simulink model "ExampleModel"  (R2019a)
settings: Solver=VariableStepAuto  StartTime=0.0  StopTime=10.0  RelTol=1e-3  EnableMultiTasking=on
values from neighbouring files (symbols this model uses):
  Param_Mus = Library_mtu_simulink_mtu_standard_parameters(Param_Mus)    [init_muscle.m]
libraries: Library_mtu_simulink x2, simulink x1
settings Model: Creator=danielhaeufle  LastModifiedBy=danielhaeufle
settings DataIOCC: ReturnWorkspaceOutputs=off
settings OptimizationCC: LifeSpan=inf
settings DebuggingCC: SFUnexpectedBacktrackingDiag=warning  SFNoUnconditionalDefaultTransitionDiag=warning  ArithmeticOperatorsInVariantConditions=warning
settings SFSimCC: SimUseLocalCustomCode=off
settings RTWCC: RTWUseLocalCustomCode=off
settings CodeAppCC: StateflowObjectComments=on
settings GRTTargetCC: TargetLangStandard=C89/C90 (ANSI)  GeneratePreprocessorConditionals=Disable all
settings ConfigComp: CovMetricSettings=dw  CovHtmlReporting=on  CovSaveCumulativeToWorkspaceVar=on  CovSaveSingleToWorkspaceVar=on  CovExternalEMLEnable=off

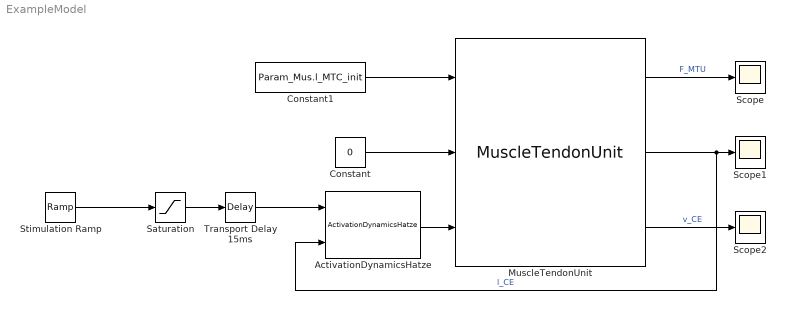
== system ExampleModel ==
  ActivationDynamicsHatze : Library_mtu_simulink/ActivationDynamicsHatze  Act_Param=Param_Mus.ActDyn  Mus_Param=Param_Mus
  Constant : Constant  Value=0
  Constant1 : Constant  Value=Param_Mus.l_MTC_init
  MuscleTendonUnit : Library_mtu_simulink/MuscleTendonUnit  Mus_Param=Param_Mus
  Saturation : Saturate  UpperLimit=1  LowerLimit=0.001
  Scope : Scope
  Scope1 : Scope
  Scope2 : Scope
  Stimulation Ramp : simulink/Sources/Ramp  slope=0.1  start=0  InitialOutput=0
  Transport Delay 15ms : TransportDelay  DelayTime=0.015  InitialOutput=Param_Mus.ActDyn.u_init
  wires:
  Saturation/1 -> Transport Delay 15ms/1
  ActivationDynamicsHatze/1 -> MuscleTendonUnit/3
  Transport Delay 15ms/1 -> ActivationDynamicsHatze/1
  Stimulation Ramp/1 -> Saturation/1
  Constant/1 -> MuscleTendonUnit/2
  Constant1/1 -> MuscleTendonUnit/1
  MuscleTendonUnit/1 -> Scope/1  "F_MTU"
  MuscleTendonUnit/2 -> ActivationDynamicsHatze/2, Scope1/1  "l_CE"
  MuscleTendonUnit/3 -> Scope2/1  "v_CE"
